simulink model "Q6"  (R2020b)
settings: Solver=VariableStepAuto  StartTime=0.0  StopTime=100.0  RelTol=1e-3
settings Model: Creator=Javad  LastModifiedBy=Javad

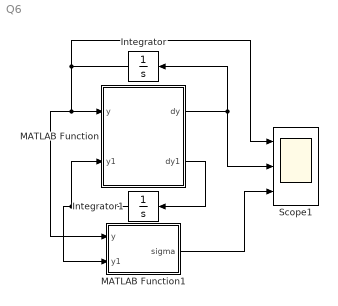
== system Q6 ==
  Integrator : Integrator  InitialCondition=1
  Integrator1 : Integrator
  MATLAB Function : MATLAB Function  TreatAsAtomicUnit=on
  MATLAB Function1 : MATLAB Function  TreatAsAtomicUnit=on
  Scope1 : Scope  NumInputPorts=3
  wires:
  MATLAB Function/1(dy) -> Integrator/1, Scope1/2
  Integrator/1 -> MATLAB Function/1(y), MATLAB Function1/1(y), Scope1/1
  MATLAB Function/2(dy1) -> Integrator1/1
  Integrator1/1 -> MATLAB Function1/2(y1), MATLAB Function/2(y1)
  MATLAB Function1/1(sigma) -> Scope1/3

== matlab function Q6/MATLAB Function ==
  data: y input; dy output; y1 input; dy1 output
function [dy,dy1] = sys(y,y1)
    dy=y1;
    dy1=y1-sign((y1+0.2*y)*y);

== matlab function Q6/MATLAB Function1 ==
  data: y input; sigma output; y1 input
function sigma = surface(y,y1)

sigma=y1+0.2*y;
